simulink model "lab3"  (R2019a)
settings: Solver=VariableStepAuto  StartTime=0.0  StopTime=10.0  RelTol=1e-3
settings Model: Creator=T.S  LastModifiedBy=T.S

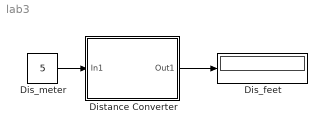
== system lab3 ==
  Dis_feet : Display
  Dis_meter : Constant  Value=5
  Distance Converter : Subsystem
  wires:
  Dis_meter/1 -> Distance Converter/1(In1)
  Distance Converter/1(Out1) -> Dis_feet/1

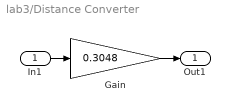
== system lab3/Distance Converter ==
  In1 : Inport
  Gain : Gain  Gain=0.3048
  Out1 : Outport
  wires:
  Gain/1 -> Out1/1
  In1/1 -> Gain/1
